simulink model "stmservo"  (R2013b)
settings: Solver=FixedStepDiscrete  StartTime=0.0  StopTime=10.0  FixedStep=sampletime  RelTol=1e-3
model workspace (MATLAB code in the model file):
  | sampletime = 0.0001;
  | pwmsampletime = 0.001;
libraries: simulink x7, stm32f4lib x5, simulink_extras x1
settings Model: Creator=Fodi  LastModifiedBy=Fodi
settings OptimizationCC: OptimizeModelRefInitCode=on  LifeSpan=1  MaxStackSize=64
settings HardwareCC: ProdLargestAtomicInteger=Long  ProdLargestAtomicFloat=Double  ProdEndianess=LittleEndian  ProdHWDeviceType=ARM Compatible->ARM Cortex
settings RTWCC: SystemTargetFile=ert.tlc  TLCOptions=-aInlineSetEventsForThisBaseRateFcn=TLC_FALSE -aSuppressMultiTaskScheduler=TLC_FALSE  TemplateMakefile=ert_default_tmf  Description=Embedded Coder  ProcessScript=ert_make_rtw_hook  Toolchain=GNU Tools for ARM Embedded Processors  BuildConfiguration=Faster Runs
settings CodeAppCC: IgnoreCustomStorageClasses=off
settings ERTTargetCC: CodeReplacementLibrary=C89/C90 (ANSI)  GenerateSampleERTMain=on  SupportNonFinite=off  SupportComplex=off  PurelyIntegerCode=on  ParenthesesLevel=Maximum

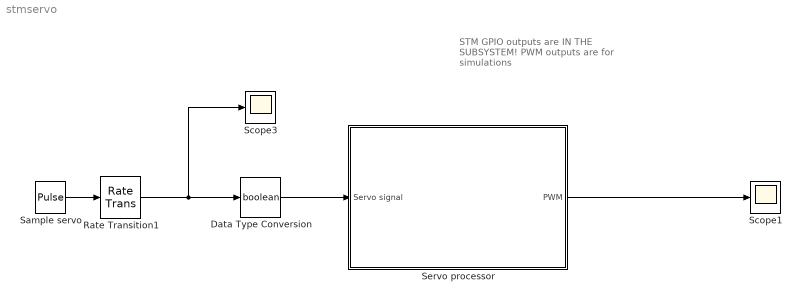
== system stmservo ==
  note: STM GPIO outputs are
      | IN THE SUBSYSTEM!
      |
      | PWM outputs are for simulations
  Data Type Conversion : DataTypeConversion  OutDataTypeStr=boolean
  Rate Transition1 : RateTransition  OutPortSampleTime=sampletime
  Sample servo : DiscretePulseGenerator  Period=200  PulseWidth=14  SampleTime=0.0001
  Scope1 : Scope
      settings: YMin=0  YMax=1.5
  Scope3 : Scope
      settings: YMin=0  YMax=1.5  SaveName=ScopeData3
  Servo processor : Subsystem
  wires:
  Sample servo/1 -> Rate Transition1/1
  Data Type Conversion/1 -> Servo processor/1(Servo signal)
  Servo processor/1(PWM) -> Scope1/1
  Rate Transition1/1 -> Data Type Conversion/1, Scope3/1

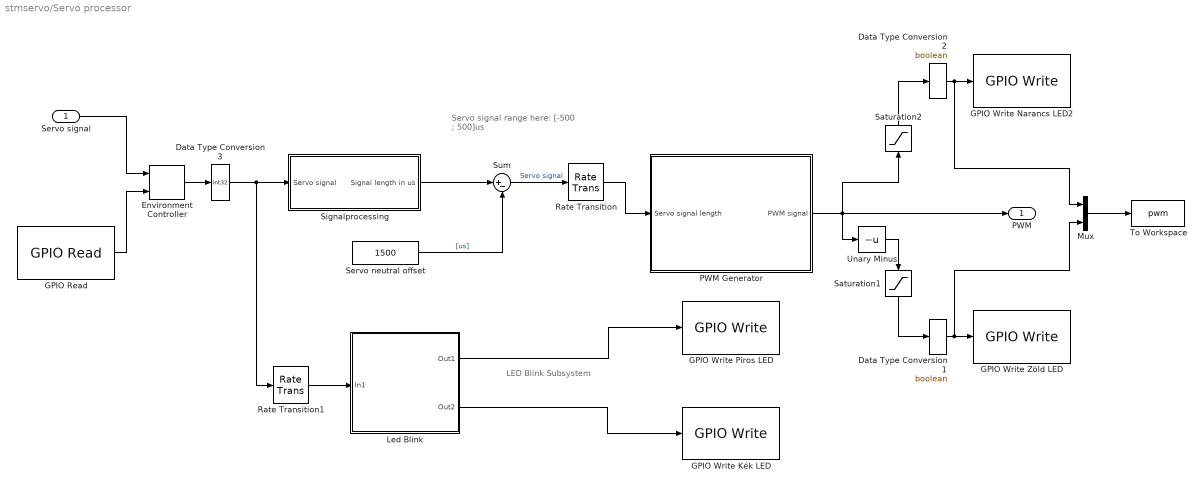
== system stmservo/Servo processor ==
  note: Servo signal range here:
      | [-500 ; 500]us
  note: LED Blink
      | Subsystem
  Servo signal : Inport
  Data Type Conversion1 : DataTypeConversion  OutDataTypeStr=boolean
  Data Type Conversion2 : DataTypeConversion  OutDataTypeStr=boolean
  Data Type Conversion3 : DataTypeConversion  OutDataTypeStr=int32
  Environment Controller : simulink/Signal Routing/Environment Controller
  GPIO Read : stm32f4lib/GPIO Read  gpio_name=GPIOB  pin_number=8  sample_time=-1  pupd_reg=0  otype_reg=0  ospeed_reg=0
  GPIO Write Kék LED : stm32f4lib/GPIO Write  gpio_name=GPIOD  pin_number=15  pupd_reg=0  otype_reg=0  ospeed_reg=0  gpio_init_out=on  toggle_pin=off
  GPIO Write Narancs LED2 : stm32f4lib/GPIO Write  gpio_name=GPIOD  pin_number=13  pupd_reg=0  otype_reg=0  ospeed_reg=0  gpio_init_out=on  toggle_pin=off
  GPIO Write Piros LED : stm32f4lib/GPIO Write  gpio_name=GPIOD  pin_number=14  pupd_reg=0  otype_reg=0  ospeed_reg=0  gpio_init_out=on  toggle_pin=off
  GPIO Write Zöld LED : stm32f4lib/GPIO Write  gpio_name=GPIOD  pin_number=12  pupd_reg=0  otype_reg=0  ospeed_reg=0  gpio_init_out=on  toggle_pin=off
  Led Blink : Subsystem  TreatAsAtomicUnit=on  SystemSampleTime=0.1
  Mux : Mux  Inputs=2
  PWM Generator : Subsystem  TreatAsAtomicUnit=on  SystemSampleTime=pwmsampletime
  Rate Transition : RateTransition
  Rate Transition1 : RateTransition  OutPortSampleTime=0.1
  Saturation1 : Saturate  UpperLimit=1  LowerLimit=0
  Saturation2 : Saturate  UpperLimit=1  LowerLimit=0
  Servo neutral offset : Constant  Value=1500  OutDataTypeStr=int32
  Signalprocessing : Subsystem
  Sum : Sum  Inputs=|+-
  To Workspace : ToWorkspace  VariableName=pwm  SampleTime=-1  SaveFormat=Timeseries
  Unary Minus : UnaryMinus
  PWM : Outport
  wires:
  Servo signal/1 -> Environment Controller/1
  Servo neutral offset/1 -> Sum/2  "[us]"
  Signalprocessing/1(Signal length in us) -> Sum/1
  Sum/1 -> Rate Transition/1  "Servo signal"
  Rate Transition/1 -> PWM Generator/1(Servo signal length)
  Unary Minus/1 -> Saturation1/1
  Saturation1/1 -> Data Type Conversion1/1
  Saturation2/1 -> Data Type Conversion2/1
  Environment Controller/1 -> Data Type Conversion3/1
  GPIO Read/1 -> Environment Controller/2
  Data Type Conversion1/1 -> Mux/2, GPIO Write Zöld LED/1
  Data Type Conversion2/1 -> Mux/1, GPIO Write Narancs LED2/1
  PWM Generator/1(PWM signal) -> Unary Minus/1, Saturation2/1, PWM/1
  Data Type Conversion3/1 -> Rate Transition1/1, Signalprocessing/1(Servo signal)
  Led Blink/1(Out1) -> GPIO Write Piros LED/1
  Led Blink/2(Out2) -> GPIO Write Kék LED/1
  Rate Transition1/1 -> Led Blink/1(In1)
  Mux/1 -> To Workspace/1

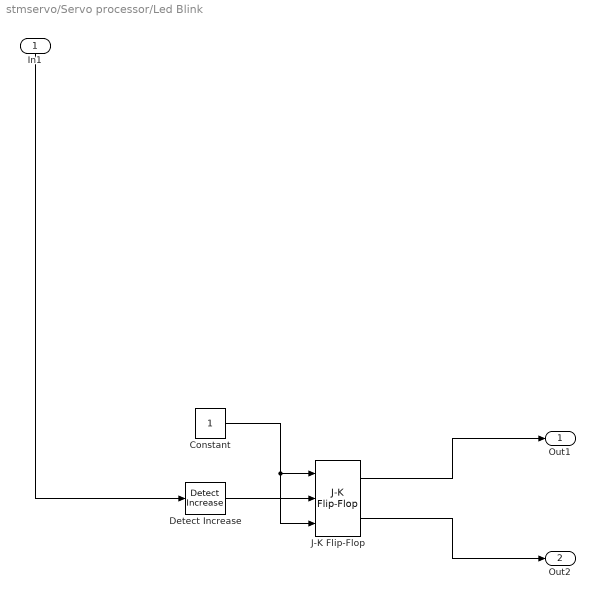
== system stmservo/Servo processor/Led Blink ==
  In1 : Inport
  Constant : Constant  OutDataTypeStr=boolean
  Detect Increase : simulink/Logic and Bit Operations/Detect Increase  vinit=0.0  InputProcessing=Inherited  OutDataTypeStr=boolean
  J-K Flip-Flop : simulink_extras/Flip Flops/J-K Flip-Flop  initial_condition=0
  Out1 : Outport
  Out2 : Outport  Port=2
  wires:
  In1/1 -> Detect Increase/1
  Constant/1 -> J-K Flip-Flop/3, J-K Flip-Flop/1
  J-K Flip-Flop/1 -> Out1/1
  Detect Increase/1 -> J-K Flip-Flop/2
  J-K Flip-Flop/2 -> Out2/1

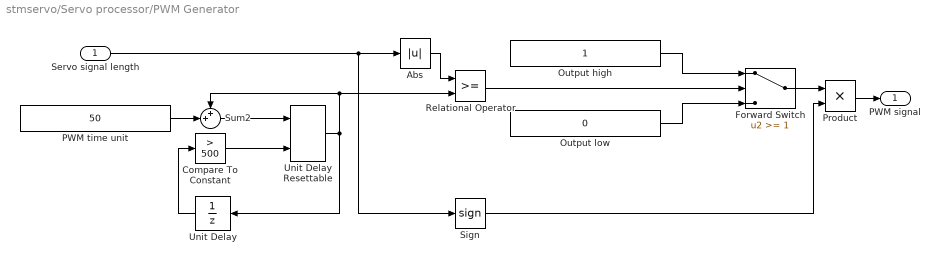
== system stmservo/Servo processor/PWM Generator ==
  Servo signal length : Inport
  Abs : Abs
  Compare To Constant : simulink/Logic and Bit Operations/Compare To Constant  relop=>  const=500  OutDataTypeStr=boolean
  Forward Switch : Switch  Threshold=1
  Output high : Constant  OutDataTypeStr=int32
  Output low : Constant  Value=0  OutDataTypeStr=int32
  PWM time unit : Constant  Value=50  OutDataTypeStr=int32
  Product : Product  OutDataTypeStr=int32
  Relational Operator : RelationalOperator  OutDataTypeStr=boolean
  Sign : Signum
  Sum2 : Sum  Inputs=++|
  Unit Delay : UnitDelay  SampleTime=-1
  Unit Delay Resettable : simulink/Additional Math & Discrete/Additional Discrete/Unit Delay Resettable  vinit=0.0  tsamp=-1
  PWM signal : Outport  OutDataTypeStr=int32
  wires:
  Sum2/1 -> Unit Delay Resettable/1
  Servo signal length/1 -> Sign/1, Abs/1
  Compare To Constant/1 -> Unit Delay Resettable/2
  Unit Delay Resettable/1 -> Relational Operator/2, Sum2/1, Unit Delay/1
  PWM time unit/1 -> Sum2/2
  Relational Operator/1 -> Forward Switch/2
  Output high/1 -> Forward Switch/1
  Output low/1 -> Forward Switch/3
  Forward Switch/1 -> Product/1
  Product/1 -> PWM signal/1
  Sign/1 -> Product/2
  Unit Delay/1 -> Compare To Constant/1
  Abs/1 -> Relational Operator/1

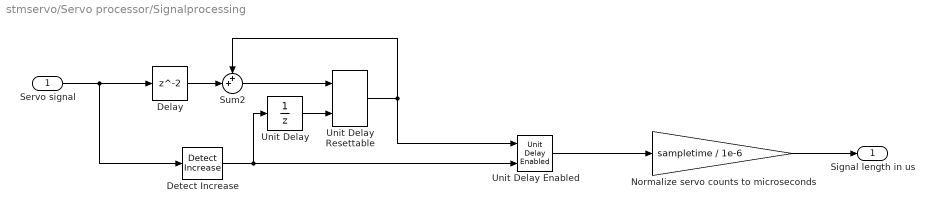
== system stmservo/Servo processor/Signalprocessing ==
  Servo signal : Inport
  Delay : Delay
  Detect Increase : simulink/Logic and Bit Operations/Detect Increase  vinit=0.0  InputProcessing=Inherited  OutDataTypeStr=boolean
  Normalize servo counts to microseconds : Gain  Gain=sampletime / 1e-6  OutDataTypeStr=int32
  Sum2 : Sum  Inputs=++|  AccumDataTypeStr=int32
  Unit Delay : UnitDelay  SampleTime=-1
  Unit Delay Enabled : simulink/Additional Math & Discrete/Additional Discrete/Unit Delay Enabled  vinit=0.0  tsamp=-1
  Unit Delay Resettable : simulink/Additional Math & Discrete/Additional Discrete/Unit Delay Resettable  vinit=0.0  tsamp=-1
  Signal length in us : Outport
  wires:
  Servo signal/1 -> Delay/1, Detect Increase/1
  Unit Delay Resettable/1 -> Unit Delay Enabled/1, Sum2/1
  Detect Increase/1 -> Unit Delay Enabled/2, Unit Delay/1
  Normalize servo counts to microseconds/1 -> Signal length in us/1
  Unit Delay Enabled/1 -> Normalize servo counts to microseconds/1
  Unit Delay/1 -> Unit Delay Resettable/2
  Sum2/1 -> Unit Delay Resettable/1
  Delay/1 -> Sum2/2
